simulink model "4_PE"  (R2015b)
settings: Solver=FixedStepDiscrete  SolverMode=SingleTasking  StartTime=0.0  StopTime=2.5e-6  RelTol=1e-3
libraries: shlslibv1 x156
settings Model: synDspstartup=OK  Creator=amitra5  LastModifiedBy=sjparekh
settings DataIOCC: SaveFormat=Array  SaveOutput=off  SignalLogging=off  SaveTime=off
settings OptimizationCC: DefaultParameterBehavior=Inlined
settings DebuggingCC: AlgebraicLoopMsg=error  SolverPrmCheckMsg=warning  InheritedTsInSrcMsg=none
settings HardwareCC: ProdBitPerPointer=32  ProdLargestAtomicFloat=None  ProdIntDivRoundTo=Undefined  ProdEndianess=Unspecified  ProdWordSize=32  ProdHWDeviceType=32-bit Generic
settings GRTTargetCC: GeneratePreprocessorConditionals=Disable all
settings ConfigComp: CovModelRefEnable=Off  CovSFcnEnable=off

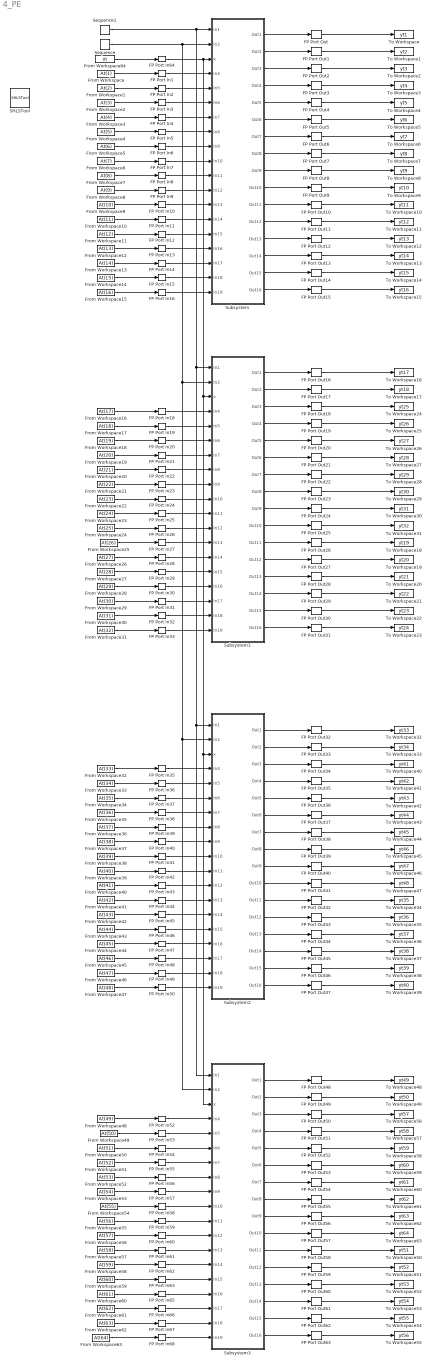
== system 4_PE ==
  FP Port In{1..16,18..33,35..50,52..68} (65 alike) : shlslibv1/Floating Point/FP Port In  synBlockType=custom  synLatency=1  syn_exp_wl=11  syn_frac_wl=52  syn_out_st=1/(504.96e6)  syn_capture=on  syn_register=on  syn_opt_ports=off
  FP Port Out{,1..63} (64 alike) : shlslibv1/Floating Point/FP Port Out  synBlockType=custom  synLatency=1  syn_exp_wl=11  syn_frac_wl=52  syn_capture=on  syn_register=on
  From Workspace : FromWorkspace  VariableName=At(1)
  From Workspace1 : FromWorkspace  VariableName=At(2)
  From Workspace10 : FromWorkspace  VariableName=At(11)
  From Workspace11 : FromWorkspace  VariableName=At(12)
  From Workspace12 : FromWorkspace  VariableName=At(13)
  From Workspace13 : FromWorkspace  VariableName=At(14)
  From Workspace14 : FromWorkspace  VariableName=At(15)
  From Workspace15 : FromWorkspace  VariableName=At(16)
  From Workspace16 : FromWorkspace  VariableName=At(17)
  From Workspace17 : FromWorkspace  VariableName=At(18)
  From Workspace18 : FromWorkspace  VariableName=At(19)
  From Workspace19 : FromWorkspace  VariableName=At(20)
  From Workspace2 : FromWorkspace  VariableName=At(3)
  From Workspace20 : FromWorkspace  VariableName=At(21)
  From Workspace21 : FromWorkspace  VariableName=At(22)
  From Workspace22 : FromWorkspace  VariableName=At(23)
  From Workspace23 : FromWorkspace  VariableName=At(24)
  From Workspace24 : FromWorkspace  VariableName=At(25)
  From Workspace25 : FromWorkspace  VariableName=At(26)
  From Workspace26 : FromWorkspace  VariableName=At(27)
  From Workspace27 : FromWorkspace  VariableName=At(28)
  From Workspace28 : FromWorkspace  VariableName=At(29)
  From Workspace29 : FromWorkspace  VariableName=At(30)
  From Workspace3 : FromWorkspace  VariableName=At(4)
  From Workspace30 : FromWorkspace  VariableName=At(31)
  From Workspace31 : FromWorkspace  VariableName=At(32)
  From Workspace32 : FromWorkspace  VariableName=At(33)
  From Workspace33 : FromWorkspace  VariableName=At(34)
  From Workspace34 : FromWorkspace  VariableName=At(35)
  From Workspace35 : FromWorkspace  VariableName=At(36)
  From Workspace36 : FromWorkspace  VariableName=At(37)
  From Workspace37 : FromWorkspace  VariableName=At(38)
  From Workspace38 : FromWorkspace  VariableName=At(39)
  From Workspace39 : FromWorkspace  VariableName=At(40)
  From Workspace4 : FromWorkspace  VariableName=At(5)
  From Workspace40 : FromWorkspace  VariableName=At(41)
  From Workspace41 : FromWorkspace  VariableName=At(42)
  From Workspace42 : FromWorkspace  VariableName=At(43)
  From Workspace43 : FromWorkspace  VariableName=At(44)
  From Workspace44 : FromWorkspace  VariableName=At(45)
  From Workspace45 : FromWorkspace  VariableName=At(46)
  From Workspace46 : FromWorkspace  VariableName=At(47)
  From Workspace47 : FromWorkspace  VariableName=At(48)
  From Workspace48 : FromWorkspace  VariableName=At(49)
  From Workspace49 : FromWorkspace  VariableName=At(50)
  From Workspace5 : FromWorkspace  VariableName=At(6)
  From Workspace50 : FromWorkspace  VariableName=At(51)
  From Workspace51 : FromWorkspace  VariableName=At(52)
  From Workspace52 : FromWorkspace  VariableName=At(53)
  From Workspace53 : FromWorkspace  VariableName=At(54)
  From Workspace54 : FromWorkspace  VariableName=At(55)
  From Workspace55 : FromWorkspace  VariableName=At(56)
  From Workspace56 : FromWorkspace  VariableName=At(57)
  From Workspace57 : FromWorkspace  VariableName=At(58)
  From Workspace58 : FromWorkspace  VariableName=At(59)
  From Workspace59 : FromWorkspace  VariableName=At(60)
  From Workspace6 : FromWorkspace  VariableName=At(7)
  From Workspace60 : FromWorkspace  VariableName=At(61)
  From Workspace61 : FromWorkspace  VariableName=At(62)
  From Workspace62 : FromWorkspace  VariableName=At(63)
  From Workspace63 : FromWorkspace  VariableName=At(64)
  From Workspace64 : FromWorkspace  VariableName=xt  Interpolate=off  OutputAfterFinalValue=Holding final value
  From Workspace7 : FromWorkspace  VariableName=At(8)
  From Workspace8 : FromWorkspace  VariableName=At(9)
  From Workspace9 : FromWorkspace  VariableName=At(10)
  SHLSTool : shlslibv1/SHLSTool  synBlockType=tool  syn_dsp_mode=FPGA
  Sequence : shlslibv1/Sources/Sequence  syn_seq_vec=[0 1 2 3 4 5 6 7 8 9 10 11 12 13 14 15]  syn_seq_wl=4  syn_seq_fl=0  syn_seq_dt=unsigned  syn_rst_port=off  syn_en_port=off  syn_seq_st=1/(504.96e6)  synBlockType=custom  synLatency=1
  Sequence1 : shlslibv1/Sources/Sequence  syn_seq_vec=[4 5 6 7 8 9 10 11 12 13 14 15 0 1 2 3]  syn_seq_wl=4  syn_seq_fl=0  syn_seq_dt=unsigned  syn_rst_port=off  syn_en_port=off  syn_seq_st=1/(504.96e6)  synBlockType=custom  synLatency=1
  Subsystem : Subsystem
  Subsystem1 : Subsystem
  Subsystem2 : Subsystem
  Subsystem3 : Subsystem
  To Workspace : ToWorkspace  VariableName=yt1  SaveFormat=Structure With Time  SampleTime=-1
      settings: Save2DSignal=2-D array (concatenate along first dimension)
  To Workspace1 : ToWorkspace  VariableName=yt2  SaveFormat=Structure With Time  SampleTime=-1
      settings: Save2DSignal=2-D array (concatenate along first dimension)
  To Workspace10 : ToWorkspace  VariableName=yt11  SaveFormat=Structure With Time  SampleTime=-1
      settings: Save2DSignal=2-D array (concatenate along first dimension)
  To Workspace11 : ToWorkspace  VariableName=yt12  SaveFormat=Structure With Time  SampleTime=-1
  To Workspace12 : ToWorkspace  VariableName=yt13  SaveFormat=Structure With Time  SampleTime=-1
      settings: Save2DSignal=2-D array (concatenate along first dimension)
  To Workspace13 : ToWorkspace  VariableName=yt14  SaveFormat=Structure With Time  SampleTime=-1
      settings: Save2DSignal=2-D array (concatenate along first dimension)
  To Workspace14 : ToWorkspace  VariableName=yt15  SaveFormat=Structure With Time  SampleTime=-1
      settings: Save2DSignal=2-D array (concatenate along first dimension)
  To Workspace15 : ToWorkspace  VariableName=yt16  SaveFormat=Structure With Time  SampleTime=-1
  To Workspace16 : ToWorkspace  VariableName=yt17  SaveFormat=Structure With Time  SampleTime=-1
      settings: Save2DSignal=2-D array (concatenate along first dimension)
  To Workspace17 : ToWorkspace  VariableName=yt18  SaveFormat=Structure With Time  SampleTime=-1
      settings: Save2DSignal=2-D array (concatenate along first dimension)
  To Workspace18 : ToWorkspace  VariableName=yt19  SaveFormat=Structure With Time  SampleTime=-1
      settings: Save2DSignal=2-D array (concatenate along first dimension)
  To Workspace19 : ToWorkspace  VariableName=yt20  SaveFormat=Structure With Time  SampleTime=-1
  To Workspace2 : ToWorkspace  VariableName=yt3  SaveFormat=Structure With Time  SampleTime=-1
      settings: Save2DSignal=2-D array (concatenate along first dimension)
  To Workspace20 : ToWorkspace  VariableName=yt21  SaveFormat=Structure With Time  SampleTime=-1
      settings: Save2DSignal=2-D array (concatenate along first dimension)
  To Workspace21 : ToWorkspace  VariableName=yt22  SaveFormat=Structure With Time  SampleTime=-1
      settings: Save2DSignal=2-D array (concatenate along first dimension)
  To Workspace22 : ToWorkspace  VariableName=yt23  SaveFormat=Structure With Time  SampleTime=-1
      settings: Save2DSignal=2-D array (concatenate along first dimension)
  To Workspace23 : ToWorkspace  VariableName=yt24  SaveFormat=Structure With Time  SampleTime=-1
  To Workspace24 : ToWorkspace  VariableName=yt25  SaveFormat=Structure With Time  SampleTime=-1
      settings: Save2DSignal=2-D array (concatenate along first dimension)
  To Workspace25 : ToWorkspace  VariableName=yt26  SaveFormat=Structure With Time  SampleTime=-1
  To Workspace26 : ToWorkspace  VariableName=yt27  SaveFormat=Structure With Time  SampleTime=-1
      settings: Save2DSignal=2-D array (concatenate along first dimension)
  To Workspace27 : ToWorkspace  VariableName=yt28  SaveFormat=Structure With Time  SampleTime=-1
      settings: Save2DSignal=2-D array (concatenate along first dimension)
  To Workspace28 : ToWorkspace  VariableName=yt29  SaveFormat=Structure With Time  SampleTime=-1
      settings: Save2DSignal=2-D array (concatenate along first dimension)
  To Workspace29 : ToWorkspace  VariableName=yt30  SaveFormat=Structure With Time  SampleTime=-1
  To Workspace3 : ToWorkspace  VariableName=yt4  SaveFormat=Structure With Time  SampleTime=-1
  To Workspace30 : ToWorkspace  VariableName=yt31  SaveFormat=Structure With Time  SampleTime=-1
      settings: Save2DSignal=2-D array (concatenate along first dimension)
  To Workspace31 : ToWorkspace  VariableName=yt32  SaveFormat=Structure With Time  SampleTime=-1
      settings: Save2DSignal=2-D array (concatenate along first dimension)
  To Workspace32 : ToWorkspace  VariableName=yt33  SaveFormat=Structure With Time  SampleTime=-1
      settings: Save2DSignal=2-D array (concatenate along first dimension)
  To Workspace33 : ToWorkspace  VariableName=yt34  SaveFormat=Structure With Time  SampleTime=-1
      settings: Save2DSignal=2-D array (concatenate along first dimension)
  To Workspace34 : ToWorkspace  VariableName=yt35  SaveFormat=Structure With Time  SampleTime=-1
      settings: Save2DSignal=2-D array (concatenate along first dimension)
  To Workspace35 : ToWorkspace  VariableName=yt36  SaveFormat=Structure With Time  SampleTime=-1
  To Workspace36 : ToWorkspace  VariableName=yt37  SaveFormat=Structure With Time  SampleTime=-1
      settings: Save2DSignal=2-D array (concatenate along first dimension)
  To Workspace37 : ToWorkspace  VariableName=yt38  SaveFormat=Structure With Time  SampleTime=-1
      settings: Save2DSignal=2-D array (concatenate along first dimension)
  To Workspace38 : ToWorkspace  VariableName=yt39  SaveFormat=Structure With Time  SampleTime=-1
      settings: Save2DSignal=2-D array (concatenate along first dimension)
  To Workspace39 : ToWorkspace  VariableName=yt40  SaveFormat=Structure With Time  SampleTime=-1
  To Workspace4 : ToWorkspace  VariableName=yt5  SaveFormat=Structure With Time  SampleTime=-1
      settings: Save2DSignal=2-D array (concatenate along first dimension)
  To Workspace40 : ToWorkspace  VariableName=yt41  SaveFormat=Structure With Time  SampleTime=-1
      settings: Save2DSignal=2-D array (concatenate along first dimension)
  To Workspace41 : ToWorkspace  VariableName=yt42  SaveFormat=Structure With Time  SampleTime=-1
  To Workspace42 : ToWorkspace  VariableName=yt43  SaveFormat=Structure With Time  SampleTime=-1
      settings: Save2DSignal=2-D array (concatenate along first dimension)
  To Workspace43 : ToWorkspace  VariableName=yt44  SaveFormat=Structure With Time  SampleTime=-1
      settings: Save2DSignal=2-D array (concatenate along first dimension)
  To Workspace44 : ToWorkspace  VariableName=yt45  SaveFormat=Structure With Time  SampleTime=-1
      settings: Save2DSignal=2-D array (concatenate along first dimension)
  To Workspace45 : ToWorkspace  VariableName=yt46  SaveFormat=Structure With Time  SampleTime=-1
  To Workspace46 : ToWorkspace  VariableName=yt47  SaveFormat=Structure With Time  SampleTime=-1
      settings: Save2DSignal=2-D array (concatenate along first dimension)
  To Workspace47 : ToWorkspace  VariableName=yt48  SaveFormat=Structure With Time  SampleTime=-1
      settings: Save2DSignal=2-D array (concatenate along first dimension)
  To Workspace48 : ToWorkspace  VariableName=yt49  SaveFormat=Structure With Time  SampleTime=-1
      settings: Save2DSignal=2-D array (concatenate along first dimension)
  To Workspace49 : ToWorkspace  VariableName=yt50  SaveFormat=Structure With Time  SampleTime=-1
      settings: Save2DSignal=2-D array (concatenate along first dimension)
  To Workspace5 : ToWorkspace  VariableName=yt6  SaveFormat=Structure With Time  SampleTime=-1
      settings: Save2DSignal=2-D array (concatenate along first dimension)
  To Workspace50 : ToWorkspace  VariableName=yt51  SaveFormat=Structure With Time  SampleTime=-1
      settings: Save2DSignal=2-D array (concatenate along first dimension)
  To Workspace51 : ToWorkspace  VariableName=yt52  SaveFormat=Structure With Time  SampleTime=-1
  To Workspace52 : ToWorkspace  VariableName=yt53  SaveFormat=Structure With Time  SampleTime=-1
      settings: Save2DSignal=2-D array (concatenate along first dimension)
  To Workspace53 : ToWorkspace  VariableName=yt54  SaveFormat=Structure With Time  SampleTime=-1
      settings: Save2DSignal=2-D array (concatenate along first dimension)
  To Workspace54 : ToWorkspace  VariableName=yt55  SaveFormat=Structure With Time  SampleTime=-1
      settings: Save2DSignal=2-D array (concatenate along first dimension)
  To Workspace55 : ToWorkspace  VariableName=yt56  SaveFormat=Structure With Time  SampleTime=-1
  To Workspace56 : ToWorkspace  VariableName=yt57  SaveFormat=Structure With Time  SampleTime=-1
      settings: Save2DSignal=2-D array (concatenate along first dimension)
  To Workspace57 : ToWorkspace  VariableName=yt58  SaveFormat=Structure With Time  SampleTime=-1
  To Workspace58 : ToWorkspace  VariableName=yt59  SaveFormat=Structure With Time  SampleTime=-1
      settings: Save2DSignal=2-D array (concatenate along first dimension)
  To Workspace59 : ToWorkspace  VariableName=yt60  SaveFormat=Structure With Time  SampleTime=-1
      settings: Save2DSignal=2-D array (concatenate along first dimension)
  To Workspace6 : ToWorkspace  VariableName=yt7  SaveFormat=Structure With Time  SampleTime=-1
      settings: Save2DSignal=2-D array (concatenate along first dimension)
  To Workspace60 : ToWorkspace  VariableName=yt61  SaveFormat=Structure With Time  SampleTime=-1
      settings: Save2DSignal=2-D array (concatenate along first dimension)
  To Workspace61 : ToWorkspace  VariableName=yt62  SaveFormat=Structure With Time  SampleTime=-1
  To Workspace62 : ToWorkspace  VariableName=yt63  SaveFormat=Structure With Time  SampleTime=-1
      settings: Save2DSignal=2-D array (concatenate along first dimension)
  To Workspace63 : ToWorkspace  VariableName=yt64  SaveFormat=Structure With Time  SampleTime=-1
      settings: Save2DSignal=2-D array (concatenate along first dimension)
  To Workspace7 : ToWorkspace  VariableName=yt8  SaveFormat=Structure With Time  SampleTime=-1
  To Workspace8 : ToWorkspace  VariableName=yt9  SaveFormat=Structure With Time  SampleTime=-1
      settings: Save2DSignal=2-D array (concatenate along first dimension)
  To Workspace9 : ToWorkspace  VariableName=yt10  SaveFormat=Structure With Time  SampleTime=-1
      settings: Save2DSignal=2-D array (concatenate along first dimension)
  wires:
  FP Port Out1/1 -> To Workspace1/1
  FP Port Out2/1 -> To Workspace2/1
  FP Port Out3/1 -> To Workspace3/1
  FP Port Out4/1 -> To Workspace4/1
  FP Port Out5/1 -> To Workspace5/1
  FP Port Out6/1 -> To Workspace6/1
  FP Port Out7/1 -> To Workspace7/1
  FP Port Out8/1 -> To Workspace8/1
  FP Port Out9/1 -> To Workspace9/1
  FP Port Out10/1 -> To Workspace10/1
  FP Port Out11/1 -> To Workspace11/1
  FP Port Out12/1 -> To Workspace12/1
  FP Port Out13/1 -> To Workspace13/1
  FP Port Out14/1 -> To Workspace14/1
  FP Port Out15/1 -> To Workspace15/1
  FP Port Out/1 -> To Workspace/1
  Subsystem/1(Out1) -> FP Port Out/1
  Subsystem/2(Out2) -> FP Port Out1/1
  Subsystem/3(Out3) -> FP Port Out2/1
  Subsystem/4(Out4) -> FP Port Out3/1
  Subsystem/11(Out11) -> FP Port Out10/1
  Subsystem/12(Out12) -> FP Port Out11/1
  Subsystem/13(Out13) -> FP Port Out12/1
  Subsystem/10(Out10) -> FP Port Out9/1
  Subsystem/9(Out9) -> FP Port Out8/1
  Subsystem/8(Out8) -> FP Port Out7/1
  Subsystem/7(Out7) -> FP Port Out6/1
  Subsystem/6(Out6) -> FP Port Out5/1
  Subsystem/5(Out5) -> FP Port Out4/1
  Subsystem/16(Out16) -> FP Port Out15/1
  Subsystem/15(Out15) -> FP Port Out14/1
  Subsystem/14(Out14) -> FP Port Out13/1
  From Workspace/1 -> FP Port In1/1
  FP Port In1/1 -> Subsystem/4(In4)
  FP Port In2/1 -> Subsystem/5(In5)
  From Workspace1/1 -> FP Port In2/1
  From Workspace2/1 -> FP Port In3/1
  FP Port In3/1 -> Subsystem/6(In6)
  FP Port In4/1 -> Subsystem/7(In7)
  From Workspace3/1 -> FP Port In4/1
  From Workspace4/1 -> FP Port In5/1
  FP Port In5/1 -> Subsystem/8(In8)
  From Workspace5/1 -> FP Port In6/1
  FP Port In6/1 -> Subsystem/9(In9)
  From Workspace6/1 -> FP Port In7/1
  FP Port In7/1 -> Subsystem/10(In10)
  From Workspace7/1 -> FP Port In8/1
  FP Port In8/1 -> Subsystem/11(In11)
  From Workspace8/1 -> FP Port In9/1
  FP Port In9/1 -> Subsystem/12(In12)
  From Workspace9/1 -> FP Port In10/1
  FP Port In10/1 -> Subsystem/13(In13)
  From Workspace10/1 -> FP Port In11/1
  FP Port In11/1 -> Subsystem/14(In14)
  From Workspace11/1 -> FP Port In12/1
  FP Port In12/1 -> Subsystem/15(In15)
  From Workspace12/1 -> FP Port In13/1
  FP Port In13/1 -> Subsystem/16(In16)
  FP Port In14/1 -> Subsystem/17(In17)
  From Workspace13/1 -> FP Port In14/1
  From Workspace14/1 -> FP Port In15/1
  FP Port In15/1 -> Subsystem/18(In18)
  From Workspace15/1 -> FP Port In16/1
  FP Port In16/1 -> Subsystem/19(In19)
  FP Port Out17/1 -> To Workspace17/1
  FP Port Out18/1 -> To Workspace24/1
  FP Port Out19/1 -> To Workspace25/1
  FP Port Out20/1 -> To Workspace26/1
  FP Port Out21/1 -> To Workspace27/1
  FP Port Out22/1 -> To Workspace28/1
  FP Port Out23/1 -> To Workspace29/1
  FP Port Out24/1 -> To Workspace30/1
  FP Port Out25/1 -> To Workspace31/1
  FP Port Out26/1 -> To Workspace18/1
  FP Port Out27/1 -> To Workspace19/1
  FP Port Out28/1 -> To Workspace20/1
  FP Port Out29/1 -> To Workspace21/1
  FP Port Out30/1 -> To Workspace22/1
  FP Port Out31/1 -> To Workspace23/1
  FP Port Out16/1 -> To Workspace16/1
  Subsystem1/1(Out1) -> FP Port Out16/1
  Subsystem1/2(Out2) -> FP Port Out17/1
  Subsystem1/3(Out3) -> FP Port Out18/1
  Subsystem1/4(Out4) -> FP Port Out19/1
  Subsystem1/11(Out11) -> FP Port Out26/1
  Subsystem1/12(Out12) -> FP Port Out27/1
  Subsystem1/13(Out13) -> FP Port Out28/1
  Subsystem1/10(Out10) -> FP Port Out25/1
  Subsystem1/9(Out9) -> FP Port Out24/1
  Subsystem1/8(Out8) -> FP Port Out23/1
  Subsystem1/7(Out7) -> FP Port Out22/1
  Subsystem1/6(Out6) -> FP Port Out21/1
  Subsystem1/5(Out5) -> FP Port Out20/1
  Subsystem1/16(Out16) -> FP Port Out31/1
  Subsystem1/15(Out15) -> FP Port Out30/1
  Subsystem1/14(Out14) -> FP Port Out29/1
  From Workspace16/1 -> FP Port In18/1
  FP Port In18/1 -> Subsystem1/4(In4)
  FP Port In19/1 -> Subsystem1/5(In5)
  From Workspace17/1 -> FP Port In19/1
  From Workspace18/1 -> FP Port In20/1
  FP Port In20/1 -> Subsystem1/6(In6)
  FP Port In21/1 -> Subsystem1/7(In7)
  From Workspace19/1 -> FP Port In21/1
  From Workspace20/1 -> FP Port In22/1
  FP Port In22/1 -> Subsystem1/8(In8)
  From Workspace21/1 -> FP Port In23/1
  FP Port In23/1 -> Subsystem1/9(In9)
  From Workspace22/1 -> FP Port In24/1
  FP Port In24/1 -> Subsystem1/10(In10)
  From Workspace23/1 -> FP Port In25/1
  FP Port In25/1 -> Subsystem1/11(In11)
  From Workspace24/1 -> FP Port In26/1
  FP Port In26/1 -> Subsystem1/12(In12)
  From Workspace25/1 -> FP Port In27/1
  FP Port In27/1 -> Subsystem1/13(In13)
  From Workspace26/1 -> FP Port In28/1
  FP Port In28/1 -> Subsystem1/14(In14)
  From Workspace27/1 -> FP Port In29/1
  FP Port In29/1 -> Subsystem1/15(In15)
  From Workspace28/1 -> FP Port In30/1
  FP Port In30/1 -> Subsystem1/16(In16)
  FP Port In31/1 -> Subsystem1/17(In17)
  From Workspace29/1 -> FP Port In31/1
  From Workspace30/1 -> FP Port In32/1
  FP Port In32/1 -> Subsystem1/18(In18)
  From Workspace31/1 -> FP Port In33/1
  FP Port In33/1 -> Subsystem1/19(In19)
  FP Port Out33/1 -> To Workspace33/1
  FP Port Out34/1 -> To Workspace40/1
  FP Port Out35/1 -> To Workspace41/1
  FP Port Out36/1 -> To Workspace42/1
  FP Port Out37/1 -> To Workspace43/1
  FP Port Out38/1 -> To Workspace44/1
  FP Port Out39/1 -> To Workspace45/1
  FP Port Out40/1 -> To Workspace46/1
  FP Port Out41/1 -> To Workspace47/1
  FP Port Out42/1 -> To Workspace34/1
  FP Port Out43/1 -> To Workspace35/1
  FP Port Out44/1 -> To Workspace36/1
  FP Port Out45/1 -> To Workspace37/1
  FP Port Out46/1 -> To Workspace38/1
  FP Port Out47/1 -> To Workspace39/1
  FP Port Out32/1 -> To Workspace32/1
  Subsystem2/1(Out1) -> FP Port Out32/1
  Subsystem2/2(Out2) -> FP Port Out33/1
  Subsystem2/3(Out3) -> FP Port Out34/1
  Subsystem2/4(Out4) -> FP Port Out35/1
  Subsystem2/11(Out11) -> FP Port Out42/1
  Subsystem2/12(Out12) -> FP Port Out43/1
  Subsystem2/13(Out13) -> FP Port Out44/1
  Subsystem2/10(Out10) -> FP Port Out41/1
  Subsystem2/9(Out9) -> FP Port Out40/1
  Subsystem2/8(Out8) -> FP Port Out39/1
  Subsystem2/7(Out7) -> FP Port Out38/1
  Subsystem2/6(Out6) -> FP Port Out37/1
  Subsystem2/5(Out5) -> FP Port Out36/1
  Subsystem2/16(Out16) -> FP Port Out47/1
  Subsystem2/15(Out15) -> FP Port Out46/1
  Subsystem2/14(Out14) -> FP Port Out45/1
  From Workspace32/1 -> FP Port In35/1
  FP Port In35/1 -> Subsystem2/4(In4)
  FP Port In36/1 -> Subsystem2/5(In5)
  From Workspace33/1 -> FP Port In36/1
  From Workspace34/1 -> FP Port In37/1
  FP Port In37/1 -> Subsystem2/6(In6)
  FP Port In38/1 -> Subsystem2/7(In7)
  From Workspace35/1 -> FP Port In38/1
  From Workspace36/1 -> FP Port In39/1
  FP Port In39/1 -> Subsystem2/8(In8)
  From Workspace37/1 -> FP Port In40/1
  FP Port In40/1 -> Subsystem2/9(In9)
  From Workspace38/1 -> FP Port In41/1
  FP Port In41/1 -> Subsystem2/10(In10)
  From Workspace39/1 -> FP Port In42/1
  FP Port In42/1 -> Subsystem2/11(In11)
  From Workspace40/1 -> FP Port In43/1
  FP Port In43/1 -> Subsystem2/12(In12)
  From Workspace41/1 -> FP Port In44/1
  FP Port In44/1 -> Subsystem2/13(In13)
  From Workspace42/1 -> FP Port In45/1
  FP Port In45/1 -> Subsystem2/14(In14)
  From Workspace43/1 -> FP Port In46/1
  FP Port In46/1 -> Subsystem2/15(In15)
  From Workspace44/1 -> FP Port In47/1
  FP Port In47/1 -> Subsystem2/16(In16)
  FP Port In48/1 -> Subsystem2/17(In17)
  From Workspace45/1 -> FP Port In48/1
  From Workspace46/1 -> FP Port In49/1
  FP Port In49/1 -> Subsystem2/18(In18)
  From Workspace47/1 -> FP Port In50/1
  FP Port In50/1 -> Subsystem2/19(In19)
  FP Port Out49/1 -> To Workspace49/1
  FP Port Out50/1 -> To Workspace56/1
  FP Port Out51/1 -> To Workspace57/1
  FP Port Out52/1 -> To Workspace58/1
  FP Port Out53/1 -> To Workspace59/1
  FP Port Out54/1 -> To Workspace60/1
  FP Port Out55/1 -> To Workspace61/1
  FP Port Out56/1 -> To Workspace62/1
  FP Port Out57/1 -> To Workspace63/1
  FP Port Out58/1 -> To Workspace50/1
  FP Port Out59/1 -> To Workspace51/1
  FP Port Out60/1 -> To Workspace52/1
  FP Port Out61/1 -> To Workspace53/1
  FP Port Out62/1 -> To Workspace54/1
  FP Port Out63/1 -> To Workspace55/1
  FP Port Out48/1 -> To Workspace48/1
  Subsystem3/1(Out1) -> FP Port Out48/1
  Subsystem3/2(Out2) -> FP Port Out49/1
  Subsystem3/3(Out3) -> FP Port Out50/1
  Subsystem3/4(Out4) -> FP Port Out51/1
  Subsystem3/11(Out11) -> FP Port Out58/1
  Subsystem3/12(Out12) -> FP Port Out59/1
  Subsystem3/13(Out13) -> FP Port Out60/1
  Subsystem3/10(Out10) -> FP Port Out57/1
  Subsystem3/9(Out9) -> FP Port Out56/1
  Subsystem3/8(Out8) -> FP Port Out55/1
  Subsystem3/7(Out7) -> FP Port Out54/1
  Subsystem3/6(Out6) -> FP Port Out53/1
  Subsystem3/5(Out5) -> FP Port Out52/1
  Subsystem3/16(Out16) -> FP Port Out63/1
  Subsystem3/15(Out15) -> FP Port Out62/1
  Subsystem3/14(Out14) -> FP Port Out61/1
  From Workspace48/1 -> FP Port In52/1
  FP Port In52/1 -> Subsystem3/4(In4)
  FP Port In53/1 -> Subsystem3/5(In5)
  From Workspace49/1 -> FP Port In53/1
  From Workspace50/1 -> FP Port In54/1
  FP Port In54/1 -> Subsystem3/6(In6)
  FP Port In55/1 -> Subsystem3/7(In7)
  From Workspace51/1 -> FP Port In55/1
  From Workspace52/1 -> FP Port In56/1
  FP Port In56/1 -> Subsystem3/8(In8)
  From Workspace53/1 -> FP Port In57/1
  FP Port In57/1 -> Subsystem3/9(In9)
  From Workspace54/1 -> FP Port In58/1
  FP Port In58/1 -> Subsystem3/10(In10)
  From Workspace55/1 -> FP Port In59/1
  FP Port In59/1 -> Subsystem3/11(In11)
  From Workspace56/1 -> FP Port In60/1
  FP Port In60/1 -> Subsystem3/12(In12)
  From Workspace57/1 -> FP Port In61/1
  FP Port In61/1 -> Subsystem3/13(In13)
  From Workspace58/1 -> FP Port In62/1
  FP Port In62/1 -> Subsystem3/14(In14)
  From Workspace59/1 -> FP Port In63/1
  FP Port In63/1 -> Subsystem3/15(In15)
  From Workspace60/1 -> FP Port In65/1
  FP Port In65/1 -> Subsystem3/16(In16)
  FP Port In66/1 -> Subsystem3/17(In17)
  From Workspace61/1 -> FP Port In66/1
  From Workspace62/1 -> FP Port In67/1
  FP Port In67/1 -> Subsystem3/18(In18)
  From Workspace63/1 -> FP Port In68/1
  FP Port In68/1 -> Subsystem3/19(In19)
  From Workspace64/1 -> FP Port In64/1
  Sequence1/1 -> Subsystem1/1(In1), Subsystem3/1(In1), Subsystem2/1(In1), Subsystem/1(In1)
  Sequence/1 -> Subsystem1/2(In2), Subsystem3/2(In2), Subsystem2/2(In2), Subsystem/2(In2)
  FP Port In64/1 -> Subsystem1/3(x), Subsystem2/3(x), Subsystem3/3(x), Subsystem/3(x)

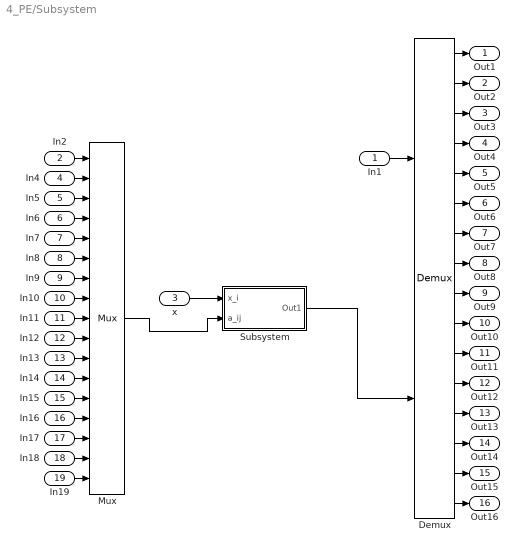
== system 4_PE/Subsystem ==
  In1 : Inport
  In2 : Inport  Port=2
  x : Inport  Port=3
  In4 : Inport  Port=4
  In5 : Inport  Port=5
  In6 : Inport  Port=6
  In7 : Inport  Port=7
  In8 : Inport  Port=8
  In9 : Inport  Port=9
  In10 : Inport  Port=10
  In11 : Inport  Port=11
  In12 : Inport  Port=12
  In13 : Inport  Port=13
  In14 : Inport  Port=14
  In15 : Inport  Port=15
  In16 : Inport  Port=16
  In17 : Inport  Port=17
  In18 : Inport  Port=18
  In19 : Inport  Port=19
  Demux : shlslibv1/Signal Operations/Demux  syn_out_nb=16  syn_out_latch=off  synBlockType=primitive  synLatency=0  synBlockId=18
  Mux : shlslibv1/Signal Operations/Mux  syn_in_nb=16  syn_out_f=Full Precision  syn_out_wl=16  syn_out_fl=8  syn_out_dt=signed  syn_en_se=off  synBlockType=primitive  synLatency=0  synBlockId=16
  Subsystem : Subsystem
  Out1 : Outport
  Out2 : Outport  Port=2
  Out3 : Outport  Port=3
  Out4 : Outport  Port=4
  Out5 : Outport  Port=5
  Out6 : Outport  Port=6
  Out7 : Outport  Port=7
  Out8 : Outport  Port=8
  Out9 : Outport  Port=9
  Out10 : Outport  Port=10
  Out11 : Outport  Port=11
  Out12 : Outport  Port=12
  Out13 : Outport  Port=13
  Out14 : Outport  Port=14
  Out15 : Outport  Port=15
  Out16 : Outport  Port=16
  wires:
  In19/1 -> Mux/17
  In18/1 -> Mux/16
  In17/1 -> Mux/15
  In16/1 -> Mux/14
  In15/1 -> Mux/13
  In14/1 -> Mux/12
  In13/1 -> Mux/11
  In12/1 -> Mux/10
  In11/1 -> Mux/9
  In10/1 -> Mux/8
  In9/1 -> Mux/7
  In8/1 -> Mux/6
  In7/1 -> Mux/5
  In6/1 -> Mux/4
  In5/1 -> Mux/3
  In4/1 -> Mux/2
  x/1 -> Subsystem/1(x_i)
  In2/1 -> Mux/1
  In1/1 -> Demux/1
  Subsystem/1(Out1) -> Demux/2
  Mux/1 -> Subsystem/2(a_ij)
  Demux/13 -> Out13/1
  Demux/12 -> Out12/1
  Demux/11 -> Out11/1
  Demux/14 -> Out14/1
  Demux/15 -> Out15/1
  Demux/16 -> Out16/1
  Demux/10 -> Out10/1
  Demux/1 -> Out1/1
  Demux/3 -> Out3/1
  Demux/2 -> Out2/1
  Demux/4 -> Out4/1
  Demux/5 -> Out5/1
  Demux/6 -> Out6/1
  Demux/7 -> Out7/1
  Demux/8 -> Out8/1
  Demux/9 -> Out9/1

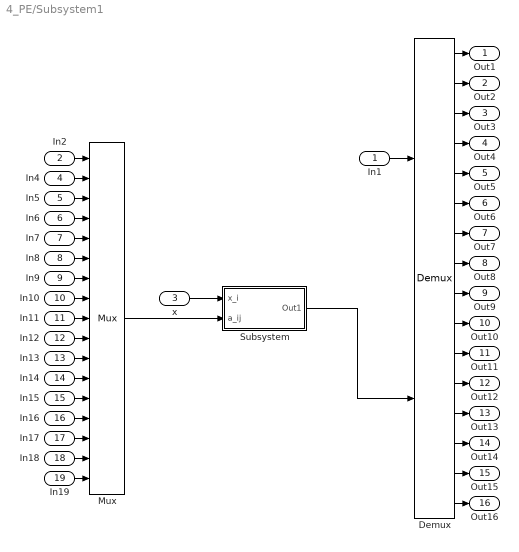
== system 4_PE/Subsystem1 ==
  In1 : Inport
  In2 : Inport  Port=2
  x : Inport  Port=3
  In4 : Inport  Port=4
  In5 : Inport  Port=5
  In6 : Inport  Port=6
  In7 : Inport  Port=7
  In8 : Inport  Port=8
  In9 : Inport  Port=9
  In10 : Inport  Port=10
  In11 : Inport  Port=11
  In12 : Inport  Port=12
  In13 : Inport  Port=13
  In14 : Inport  Port=14
  In15 : Inport  Port=15
  In16 : Inport  Port=16
  In17 : Inport  Port=17
  In18 : Inport  Port=18
  In19 : Inport  Port=19
  Demux : shlslibv1/Signal Operations/Demux  syn_out_nb=16  syn_out_latch=off  synBlockType=primitive  synLatency=0  synBlockId=18
  Mux : shlslibv1/Signal Operations/Mux  syn_in_nb=16  syn_out_f=Full Precision  syn_out_wl=16  syn_out_fl=8  syn_out_dt=signed  syn_en_se=off  synBlockType=primitive  synLatency=0  synBlockId=16
  Subsystem : Subsystem
  Out1 : Outport
  Out2 : Outport  Port=2
  Out3 : Outport  Port=3
  Out4 : Outport  Port=4
  Out5 : Outport  Port=5
  Out6 : Outport  Port=6
  Out7 : Outport  Port=7
  Out8 : Outport  Port=8
  Out9 : Outport  Port=9
  Out10 : Outport  Port=10
  Out11 : Outport  Port=11
  Out12 : Outport  Port=12
  Out13 : Outport  Port=13
  Out14 : Outport  Port=14
  Out15 : Outport  Port=15
  Out16 : Outport  Port=16
  wires:
  In19/1 -> Mux/17
  In18/1 -> Mux/16
  In17/1 -> Mux/15
  In16/1 -> Mux/14
  In15/1 -> Mux/13
  In14/1 -> Mux/12
  In13/1 -> Mux/11
  In12/1 -> Mux/10
  In11/1 -> Mux/9
  In10/1 -> Mux/8
  In9/1 -> Mux/7
  In8/1 -> Mux/6
  In7/1 -> Mux/5
  In6/1 -> Mux/4
  In5/1 -> Mux/3
  In4/1 -> Mux/2
  x/1 -> Subsystem/1(x_i)
  In2/1 -> Mux/1
  In1/1 -> Demux/1
  Subsystem/1(Out1) -> Demux/2
  Mux/1 -> Subsystem/2(a_ij)
  Demux/13 -> Out13/1
  Demux/12 -> Out12/1
  Demux/11 -> Out11/1
  Demux/14 -> Out14/1
  Demux/15 -> Out15/1
  Demux/16 -> Out16/1
  Demux/10 -> Out10/1
  Demux/1 -> Out1/1
  Demux/3 -> Out3/1
  Demux/2 -> Out2/1
  Demux/4 -> Out4/1
  Demux/5 -> Out5/1
  Demux/6 -> Out6/1
  Demux/7 -> Out7/1
  Demux/8 -> Out8/1
  Demux/9 -> Out9/1

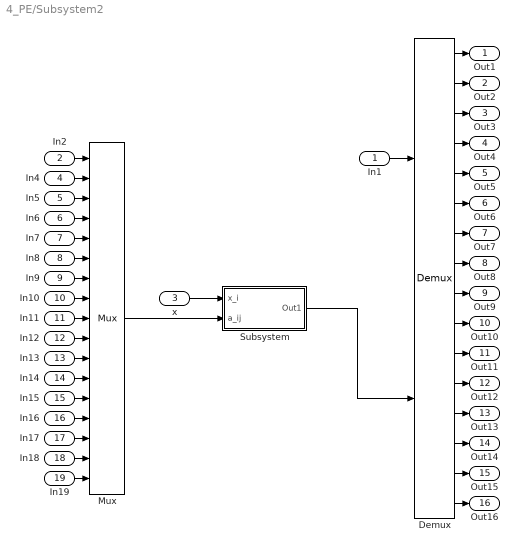
== system 4_PE/Subsystem2 ==
  In1 : Inport
  In2 : Inport  Port=2
  x : Inport  Port=3
  In4 : Inport  Port=4
  In5 : Inport  Port=5
  In6 : Inport  Port=6
  In7 : Inport  Port=7
  In8 : Inport  Port=8
  In9 : Inport  Port=9
  In10 : Inport  Port=10
  In11 : Inport  Port=11
  In12 : Inport  Port=12
  In13 : Inport  Port=13
  In14 : Inport  Port=14
  In15 : Inport  Port=15
  In16 : Inport  Port=16
  In17 : Inport  Port=17
  In18 : Inport  Port=18
  In19 : Inport  Port=19
  Demux : shlslibv1/Signal Operations/Demux  syn_out_nb=16  syn_out_latch=off  synBlockType=primitive  synLatency=0  synBlockId=18
  Mux : shlslibv1/Signal Operations/Mux  syn_in_nb=16  syn_out_f=Full Precision  syn_out_wl=16  syn_out_fl=8  syn_out_dt=signed  syn_en_se=off  synBlockType=primitive  synLatency=0  synBlockId=16
  Subsystem : Subsystem
  Out1 : Outport
  Out2 : Outport  Port=2
  Out3 : Outport  Port=3
  Out4 : Outport  Port=4
  Out5 : Outport  Port=5
  Out6 : Outport  Port=6
  Out7 : Outport  Port=7
  Out8 : Outport  Port=8
  Out9 : Outport  Port=9
  Out10 : Outport  Port=10
  Out11 : Outport  Port=11
  Out12 : Outport  Port=12
  Out13 : Outport  Port=13
  Out14 : Outport  Port=14
  Out15 : Outport  Port=15
  Out16 : Outport  Port=16
  wires:
  In19/1 -> Mux/17
  In18/1 -> Mux/16
  In17/1 -> Mux/15
  In16/1 -> Mux/14
  In15/1 -> Mux/13
  In14/1 -> Mux/12
  In13/1 -> Mux/11
  In12/1 -> Mux/10
  In11/1 -> Mux/9
  In10/1 -> Mux/8
  In9/1 -> Mux/7
  In8/1 -> Mux/6
  In7/1 -> Mux/5
  In6/1 -> Mux/4
  In5/1 -> Mux/3
  In4/1 -> Mux/2
  x/1 -> Subsystem/1(x_i)
  In2/1 -> Mux/1
  In1/1 -> Demux/1
  Subsystem/1(Out1) -> Demux/2
  Mux/1 -> Subsystem/2(a_ij)
  Demux/13 -> Out13/1
  Demux/12 -> Out12/1
  Demux/11 -> Out11/1
  Demux/14 -> Out14/1
  Demux/15 -> Out15/1
  Demux/16 -> Out16/1
  Demux/10 -> Out10/1
  Demux/1 -> Out1/1
  Demux/3 -> Out3/1
  Demux/2 -> Out2/1
  Demux/4 -> Out4/1
  Demux/5 -> Out5/1
  Demux/6 -> Out6/1
  Demux/7 -> Out7/1
  Demux/8 -> Out8/1
  Demux/9 -> Out9/1

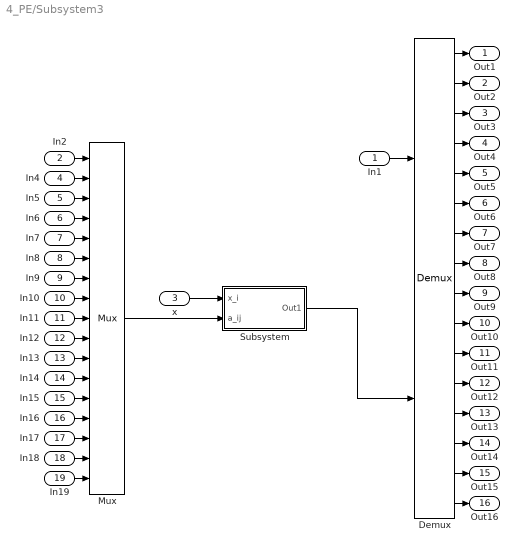
== system 4_PE/Subsystem3 ==
  In1 : Inport
  In2 : Inport  Port=2
  x : Inport  Port=3
  In4 : Inport  Port=4
  In5 : Inport  Port=5
  In6 : Inport  Port=6
  In7 : Inport  Port=7
  In8 : Inport  Port=8
  In9 : Inport  Port=9
  In10 : Inport  Port=10
  In11 : Inport  Port=11
  In12 : Inport  Port=12
  In13 : Inport  Port=13
  In14 : Inport  Port=14
  In15 : Inport  Port=15
  In16 : Inport  Port=16
  In17 : Inport  Port=17
  In18 : Inport  Port=18
  In19 : Inport  Port=19
  Demux : shlslibv1/Signal Operations/Demux  syn_out_nb=16  syn_out_latch=off  synBlockType=primitive  synLatency=0  synBlockId=18
  Mux : shlslibv1/Signal Operations/Mux  syn_in_nb=16  syn_out_f=Full Precision  syn_out_wl=16  syn_out_fl=8  syn_out_dt=signed  syn_en_se=off  synBlockType=primitive  synLatency=0  synBlockId=16
  Subsystem : Subsystem
  Out1 : Outport
  Out2 : Outport  Port=2
  Out3 : Outport  Port=3
  Out4 : Outport  Port=4
  Out5 : Outport  Port=5
  Out6 : Outport  Port=6
  Out7 : Outport  Port=7
  Out8 : Outport  Port=8
  Out9 : Outport  Port=9
  Out10 : Outport  Port=10
  Out11 : Outport  Port=11
  Out12 : Outport  Port=12
  Out13 : Outport  Port=13
  Out14 : Outport  Port=14
  Out15 : Outport  Port=15
  Out16 : Outport  Port=16
  wires:
  In19/1 -> Mux/17
  In18/1 -> Mux/16
  In17/1 -> Mux/15
  In16/1 -> Mux/14
  In15/1 -> Mux/13
  In14/1 -> Mux/12
  In13/1 -> Mux/11
  In12/1 -> Mux/10
  In11/1 -> Mux/9
  In10/1 -> Mux/8
  In9/1 -> Mux/7
  In8/1 -> Mux/6
  In7/1 -> Mux/5
  In6/1 -> Mux/4
  In5/1 -> Mux/3
  In4/1 -> Mux/2
  x/1 -> Subsystem/1(x_i)
  In2/1 -> Mux/1
  In1/1 -> Demux/1
  Subsystem/1(Out1) -> Demux/2
  Mux/1 -> Subsystem/2(a_ij)
  Demux/13 -> Out13/1
  Demux/12 -> Out12/1
  Demux/11 -> Out11/1
  Demux/14 -> Out14/1
  Demux/15 -> Out15/1
  Demux/16 -> Out16/1
  Demux/10 -> Out10/1
  Demux/1 -> Out1/1
  Demux/3 -> Out3/1
  Demux/2 -> Out2/1
  Demux/4 -> Out4/1
  Demux/5 -> Out5/1
  Demux/6 -> Out6/1
  Demux/7 -> Out7/1
  Demux/8 -> Out8/1
  Demux/9 -> Out9/1

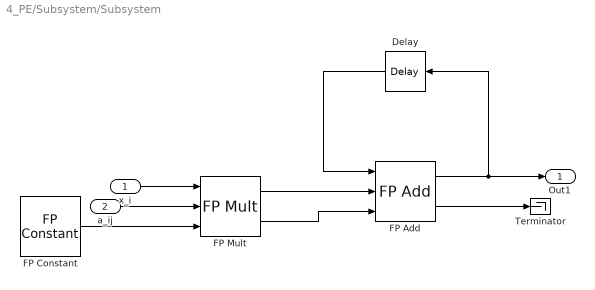
== system 4_PE/Subsystem/Subsystem ==
  x_i : Inport
  a_ij : Inport  Port=2
  Delay : shlslibv1/Memories/Delay  syn_delay_val=7  synBlockType=primitive  synLatency=7  synBlockId=104
  FP Add : shlslibv1/Floating Point/FP Add  syn_exp_wl=11  syn_frac_wl=52  syn_opt_ports=off  syn_add_opr=add  synBlockType=custom  synLatency=9
  FP Constant : shlslibv1/Floating Point/FP Constant  syn_constant_val=1  syn_exp_wl=11  syn_frac_wl=52  syn_cst_st=1/504.96e6  synBlockType=custom  synLatency=0
  FP Mult : shlslibv1/Floating Point/FP Mult  syn_exp_wl=11  syn_frac_wl=52  syn_opt_ports=off  synBlockType=custom  synLatency=3  syn_opt_tar=Default  syn_fracmult_pipe=1
  Terminator : Terminator
  Out1 : Outport
  wires:
  FP Constant/1 -> FP Mult/3
  x_i/1 -> FP Mult/1
  a_ij/1 -> FP Mult/2
  FP Add/1 -> Delay/1, Out1/1
  FP Add/2 -> Terminator/1
  FP Mult/1 -> FP Add/2
  FP Mult/2 -> FP Add/3
  Delay/1 -> FP Add/1

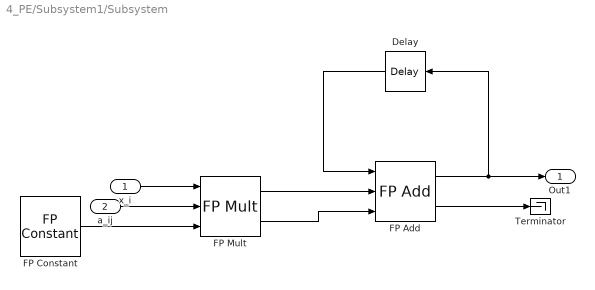
== system 4_PE/Subsystem1/Subsystem ==
  x_i : Inport
  a_ij : Inport  Port=2
  Delay : shlslibv1/Memories/Delay  syn_delay_val=7  synBlockType=primitive  synLatency=7  synBlockId=104
  FP Add : shlslibv1/Floating Point/FP Add  syn_exp_wl=11  syn_frac_wl=52  syn_opt_ports=off  syn_add_opr=add  synBlockType=custom  synLatency=9
  FP Constant : shlslibv1/Floating Point/FP Constant  syn_constant_val=1  syn_exp_wl=11  syn_frac_wl=52  syn_cst_st=1/504.96e6  synBlockType=custom  synLatency=0
  FP Mult : shlslibv1/Floating Point/FP Mult  syn_exp_wl=11  syn_frac_wl=52  syn_opt_ports=off  synBlockType=custom  synLatency=3  syn_opt_tar=Default  syn_fracmult_pipe=1
  Terminator : Terminator
  Out1 : Outport
  wires:
  FP Constant/1 -> FP Mult/3
  x_i/1 -> FP Mult/1
  a_ij/1 -> FP Mult/2
  FP Add/1 -> Delay/1, Out1/1
  FP Add/2 -> Terminator/1
  FP Mult/1 -> FP Add/2
  FP Mult/2 -> FP Add/3
  Delay/1 -> FP Add/1

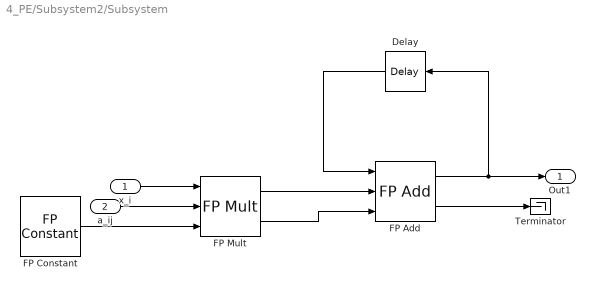
== system 4_PE/Subsystem2/Subsystem ==
  x_i : Inport
  a_ij : Inport  Port=2
  Delay : shlslibv1/Memories/Delay  syn_delay_val=7  synBlockType=primitive  synLatency=7  synBlockId=104
  FP Add : shlslibv1/Floating Point/FP Add  syn_exp_wl=11  syn_frac_wl=52  syn_opt_ports=off  syn_add_opr=add  synBlockType=custom  synLatency=9
  FP Constant : shlslibv1/Floating Point/FP Constant  syn_constant_val=1  syn_exp_wl=11  syn_frac_wl=52  syn_cst_st=1/504.96e6  synBlockType=custom  synLatency=0
  FP Mult : shlslibv1/Floating Point/FP Mult  syn_exp_wl=11  syn_frac_wl=52  syn_opt_ports=off  synBlockType=custom  synLatency=3  syn_opt_tar=Default  syn_fracmult_pipe=1
  Terminator : Terminator
  Out1 : Outport
  wires:
  FP Constant/1 -> FP Mult/3
  x_i/1 -> FP Mult/1
  a_ij/1 -> FP Mult/2
  FP Add/1 -> Delay/1, Out1/1
  FP Add/2 -> Terminator/1
  FP Mult/1 -> FP Add/2
  FP Mult/2 -> FP Add/3
  Delay/1 -> FP Add/1

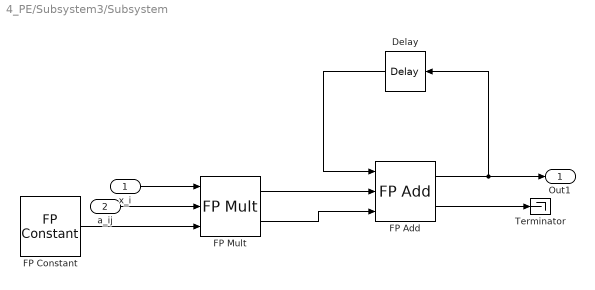
== system 4_PE/Subsystem3/Subsystem ==
  x_i : Inport
  a_ij : Inport  Port=2
  Delay : shlslibv1/Memories/Delay  syn_delay_val=7  synBlockType=primitive  synLatency=7  synBlockId=104
  FP Add : shlslibv1/Floating Point/FP Add  syn_exp_wl=11  syn_frac_wl=52  syn_opt_ports=off  syn_add_opr=add  synBlockType=custom  synLatency=9
  FP Constant : shlslibv1/Floating Point/FP Constant  syn_constant_val=1  syn_exp_wl=11  syn_frac_wl=52  syn_cst_st=1/504.96e6  synBlockType=custom  synLatency=0
  FP Mult : shlslibv1/Floating Point/FP Mult  syn_exp_wl=11  syn_frac_wl=52  syn_opt_ports=off  synBlockType=custom  synLatency=3  syn_opt_tar=Default  syn_fracmult_pipe=1
  Terminator : Terminator
  Out1 : Outport
  wires:
  FP Constant/1 -> FP Mult/3
  x_i/1 -> FP Mult/1
  a_ij/1 -> FP Mult/2
  FP Add/1 -> Delay/1, Out1/1
  FP Add/2 -> Terminator/1
  FP Mult/1 -> FP Add/2
  FP Mult/2 -> FP Add/3
  Delay/1 -> FP Add/1
